simulink model "KalmanGyro"  (R2018a)
settings: Solver=VariableStepAuto  StartTime=0.0  StopTime=10.0  RelTol=1e-3
undefined symbols (not defined in the file or in its folder): Continuous, Gssd, Time
libraries: ctrlSharedLib x1
settings Model: Creator=Philip  LastModifiedBy=Philip

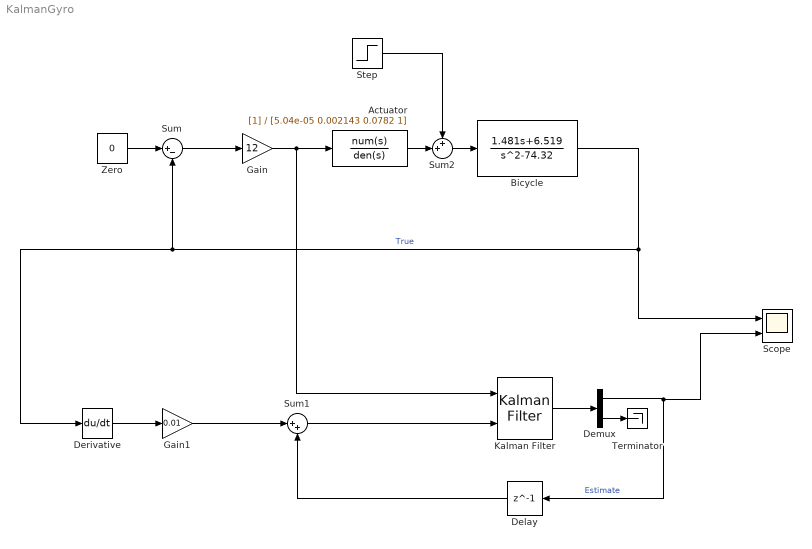
== system KalmanGyro ==
  Actuator : TransferFcn  Denominator=[5.04e-05 0.002143 0.0782 1]
  Bicycle : TransferFcn  Numerator=[1.481 6.519]  Denominator=[1 0 -74.32]
  Delay : Delay  DelayLength=1
  Demux : Demux  Outputs=2
  Derivative : Derivative  CoefficientInTFapproximation=0.001
  Gain : Gain  Gain=12
  Gain1 : Gain  Gain=0.01
  Kalman Filter : ctrlSharedLib/Kalman Filter  TimeDomain=Continuous-Time  UseCurrentEstimator=on  ModelSource=LTI State-Space Variable  ModelSourceVariable=Gss  A=Gssd  B=1  C=1  D=0  NumberOfStates=1  NumberOfInputs=1  NumberOfOutputs=1  InitialEstimateSource=Dialog  X0=0  P0=10  UseK=off  UseGH=off  NumberOfProcessNoiseInputs=1  G=1  TimeInvariantG=on  H=0  TimeInvariantH=on  Q=0.01  TimeInvariantQ=on  R=1  TimeInvariantR=on  N=0  TimeInvariantN=on  AddInputPort=on  AddEnablePort=off  OutputEstimatedY=off  OutputP=off  Ts=-1
      settings: SourceProductBaseCode=CT
  Scope : Scope  NumInputPorts=2
  Step : Step  SampleTime=0
  Sum : Sum  Inputs=|+-
  Sum1 : Sum  Inputs=|++
  Sum2 : Sum  Inputs=++|
  Terminator : Terminator
  Zero : Constant  Value=0
  wires:
  Sum/1 -> Gain/1
  Bicycle/1 -> Scope/1, Derivative/1, Sum/2  "True"
  Gain1/1 -> Sum1/1
  Delay/1 -> Sum1/2
  Kalman Filter/1 -> Demux/1
  Demux/2 -> Terminator/1
  Demux/1 -> Scope/2, Delay/1  "Estimate"
  Derivative/1 -> Gain1/1
  Gain/1 -> Kalman Filter/1, Actuator/1
  Sum1/1 -> Kalman Filter/2
  Zero/1 -> Sum/1
  Actuator/1 -> Sum2/2
  Sum2/1 -> Bicycle/1
  Step/1 -> Sum2/1
